simulink model "dc_dc_converter"  (Simulink 7.5)
settings: Solver=ode45  StartTime=0.0  StopTime=10.0  RelTol=1e-3
undefined symbols (not defined in the file): powergui
libraries: powerlib x9
settings Model: Creator=mustafasyyd  LastModifiedBy=mustafasyyd

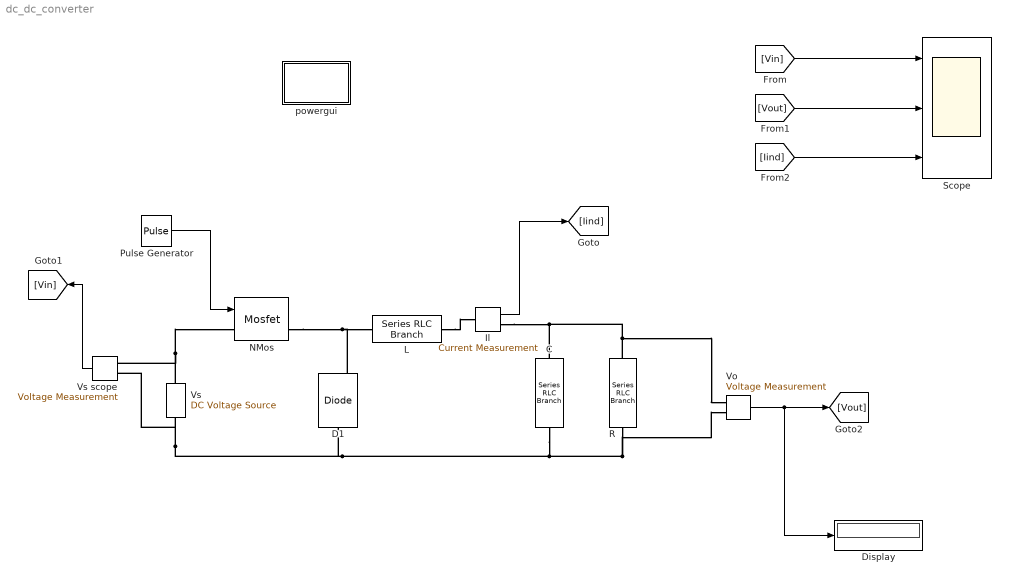
== system dc_dc_converter ==
  C : powerlib/Elements/Series RLC Branch  DialogController=POWERSYS.PowerSysDialog  PhysicalDomain=powersysdomain  SubClassName=unknown  LeftPortType=p1  RightPortType=p1  LConnTagsString=__new0  RConnTagsString=__new0  BranchType=C  Resistance=1  Inductance=1e-3  SetiL0=off  InitialCurrent=0  Capacitance=100e-6  Setx0=off  InitialVoltage=0  Measurements=None
  D1 : powerlib/Power Electronics/Diode  DialogController=POWERSYS.PowerSysDialog  SystemSampleTime=-1  Ron=0.001  Lon=0  Vf=0  IC=0  UseSnubber=off  Rs=500  Cs=250e-9  Measurements=on
  Display : Display
  Il : powerlib/Measurements/Current Measurement  DialogController=POWERSYS.PowerSysDialog  SystemSampleTime=-1  PhasorSimulation=off  OutputType=Complex  PSBequivalent=0
  L : powerlib/Elements/Series RLC Branch  DialogController=POWERSYS.PowerSysDialog  PhysicalDomain=powersysdomain  SubClassName=unknown  LeftPortType=p1  RightPortType=p1  LConnTagsString=__new0  RConnTagsString=__new0  BranchType=L  Resistance=1  Inductance=97.5e-6  SetiL0=off  InitialCurrent=0  Capacitance=1e-6  Setx0=off  InitialVoltage=0  Measurements=None
  NMos : powerlib/Power Electronics/Mosfet  DialogController=POWERSYS.PowerSysDialog  SystemSampleTime=-1  Ron=0.1  Lon=0  Rd=0.01  Vfd=0  IC=0  Rs=1e5  Cs=inf  Measurements=on
  Pulse Generator : DiscretePulseGenerator  PulseType=Time based  Amplitude=1  Period=1/40000  PulseWidth=0.375*100  PhaseDelay=0  SampleTime=1
  R : powerlib/Elements/Series RLC Branch  DialogController=POWERSYS.PowerSysDialog  PhysicalDomain=powersysdomain  SubClassName=unknown  LeftPortType=p1  RightPortType=p1  LConnTagsString=__new0  RConnTagsString=__new0  BranchType=R  Resistance=10  Inductance=0  SetiL0=off  InitialCurrent=0  Capacitance=0  Setx0=off  InitialVoltage=0  Measurements=None
  Scope : Scope  NumInputPorts=3
      settings: TimeRange=10  YMin=48~38.3575~5.55112e-017  YMax=48~38.405~1.3
  Vo : powerlib/Measurements/Voltage Measurement  DialogController=POWERSYS.PowerSysDialog  SystemSampleTime=-1  PhasorSimulation=off  OutputType=Complex  PSBequivalent=0
  Vs : powerlib/Electrical Sources/DC Voltage Source  DialogController=POWERSYS.PowerSysDialog  SystemSampleTime=-1  Amplitude=48  Measurements=None
  Vs scope : powerlib/Measurements/Voltage Measurement  DialogController=POWERSYS.PowerSysDialog  SystemSampleTime=-1  PhasorSimulation=off  OutputType=Complex  PSBequivalent=0
  powergui : Subsystem  Priority=1  AncestorBlock=powerlib/powergui  InitFcn=powergui( 'InitFcn_Callback' , gcb , 0 , [ ] );  StopFcn=powergui( 'StopFcn_Callback' , gcb , 0 , [ ] );  mask(PSB option menu block){SimulationMode=Continuous, SampleTime=50e-6, frequency=60, SPID=off, DisableSnubberDevices=off, DisableRonSwitches=off, DisableVfSwitches=off, SwTol=0, Interpol=off, frequencyindice=0, echomessages=off, HookPort=off, DisplayEquations=off, FunctionMessages=off, EnableUseOfTLC=off, x0status=blocks, RestoreLinks=warning, ResistiveCurrentMeasurement=off, Frange=, Ylog=off, Xlog=on, ShowGrid=off, save=off, variable=ZData, structure=, ZoomFFT=off, StartTime=0.0, cycles=1, DisplayStyle=1, fundamental=, FreqAxis=off, MaxFrequency=1000, frequencyindicesteady=1, RmsSteady=, display=off, Ts=, methode=off}
      mask prompts: SimulationMode "Simulation type:"; SampleTime "Sample time (s):"; frequency "Phasor frequency (Hz):"; SPID "Enable use of ideal switching devices"; DisableSnubberDevices "Disable snubbers in switching devices"; DisableRonSwitches "Disable On resistance in switching devices (Ron=0)"; DisableVfSwitches "Disable Forward voltage in switching devices (Vf=0)"; SwTol "Switch tolerance"; Interpol "Interpolate"; frequencyindice "Load flow frequency (Hz):"; echomessages "Display SimPowerSystems warnings and messages"; HookPort "Add a hook port to the powergui block"; DisplayEquations "Display circuit differential equations"; FunctionMessages "Display internal function messages (debug mode feature)"; EnableUseOfTLC "Use TLC file when in Accelerator Simulation Mode and for RTW applications"; x0status "Start simulation with initial electrical states from:"; RestoreLinks "Restore disabled links of SimPowerSystems blocks:"; ResistiveCurrentMeasurement "Use non ideal current measurement blocks (1e-4Ohm internal resistance)"; Frange "Frequency Range"; Ylog "Log impedance"; Xlog "log Frequency"; ShowGrid "grid"; save "Save Data To Workspace"; variable "Variable Name"; structure "Structure Name (PSBFFTSCOPE)"; ZoomFFT "ZoomFFT (PSBFFTSCOPE)"; StartTime "Start Time (PSBFFTSCOPE)"; cycles "Cycles (PSBFFTSCOPE)"; DisplayStyle "Display style (PSBFFTSCOPE)"; fundamental "Fundamental (PSBFFTSCOPE)"; FreqAxis "Frequency Axis (PSBFFTSCOPE)"; MaxFrequency "Max Frequency (PSBFFTSCOPE)"; frequencyindicesteady "Frequency indice (STEADYSTATE)"; RmsSteady "RMS display (STEADYSTATE)"; display "Display Results"; Ts "Old Ts setting (OBSOLETE)"; methode "Phasor simulation (OBSOLETE)"
      mask help: Set simulation type, simulation parameters, and preferences
      mask init:
      | message = powergui('MaskInitialization',gcb,SimulationMode,SampleTime);
      settings: CopyFcn=powergui( 'Copy_Callback' , gcb , 0 , [ ] );  ModelCloseFcn=powergui( 'CloseButton_Callback' , gcb , [ ] , [ ] );  NameChangeFcn=powergui( 'NameChangeFcn_Callback' , gcb , 0 , [ ] );  OpenFcn=powergui(gcb,'Open')
      settings: DeleteFcn=|
      | powergui( 'Copy_Callback' , gcb , 1 , [ ] );
      | powergui( 'CloseButton_Callback' , gcb , [ ] , [ ] );
      settings: PreSaveFcn=|
      | powergui( 'PreSaveFcn_Callback' , gcb , [ ] , [ ] );
      | powergui( 'CloseButton_Callback' , gcb , [ ] , [ ] );
      mask Help: web(psbhelp)
      mask StyleString: popup(Continuous|Discrete|Phasor),edit,edit,checkbox,checkbox,checkbox,checkbox,edit,checkbox,edit,checkbox,checkbox,checkbox,checkbox,checkbox,popup(blocks|steady|zero),popup(yes|warning|no),checkbox,edit,checkbox,checkbox,checkbox,checkbox,edit,edit,checkbox,edit,edit,edit,edit,checkbox,edit,edit,edit,checkbox,edit,checkbox
      mask CallbackString: powergui('SimulationType',[],[],gcb);|||powergui('SPID',[],[],gcb);||||||||powergui('HookPort',[],[],gcb);|||||||||||||||||||||||||
      mask TabNameString: Solver,Solver,Solver,Solver,Solver,Solver,Solver,Solver,Solver,Preferences,Preferences,Preferences,Solver,Solver,Preferences,Preferences,Preferences,Preferences,Preferences,Preferences,Preferences,Preferences,Preferences,Preferences,Preferences,Preferences,Preferences,Preferences,Preferences,Preferences,Preferences,Preferences,Preferences,Preferences,Preferences,Solver,Solver
      mask Display: color('blue'),disp(message)
  wires:
  Il/1 -> [Iind]
  Pulse Generator/1 -> NMos/1
  Vo/1 -> Display/1, [Vout]
  Vs scope/1 -> [Vin]
  [Iind] -> Scope/3
  [Vout] -> Scope/2
  [Vin] -> Scope/1
  connections:
  R/LConn1 -- C/LConn1 -- Il/RConn1 -- Vo/LConn1
  NMos/RConn1 -- L/LConn1 -- D1/RConn1
  Vs/RConn1 -- NMos/LConn1 -- Vs scope/LConn1
  L/RConn1 -- Il/LConn1
  C/RConn1 -- R/RConn1 -- Vo/LConn2 -- D1/LConn1 -- Vs/LConn1 -- Vs scope/LConn2

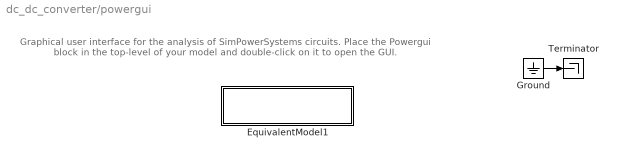
== system dc_dc_converter/powergui ==
  note: Graphical user interface for the analysis of  SimPowerSystems circuits.
      | Place the Powergui block in the top-level of your model and double-click
      | on it to open the GUI.
  EquivalentModel1 : Subsystem
      mask init:
      | S  = GetDataForEquivalentModel('Continuous',gcbh);
      mask Display:
      | color('blue')
      | disp('EQUIVALENT CIRCUIT\nContinuous')
      | disp('')
  Ground : Ground
  Terminator : Terminator
  wires:
  Ground/1 -> Terminator/1

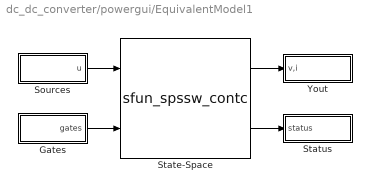
== system dc_dc_converter/powergui/EquivalentModel1 ==
  Gates : Subsystem
  Sources : Subsystem
  State-Space : S-Function  FunctionName=sfun_spssw_contc  Parameters=S.A, S.B, S.C, S.D, S.x0, S.EnableUseOfTLC,S.SwitchResistance ,S.SwitchType, S.SwitchGateInitialValue, S.OutputsToResetToZero  EnableBusSupport=off
  Status : Subsystem
  Yout : Subsystem
  wires:
  Gates/1(gates) -> State-Space/2
  Sources/1(u) -> State-Space/1
  State-Space/2 -> Status/1(status)
  State-Space/1 -> Yout/1(v,i)

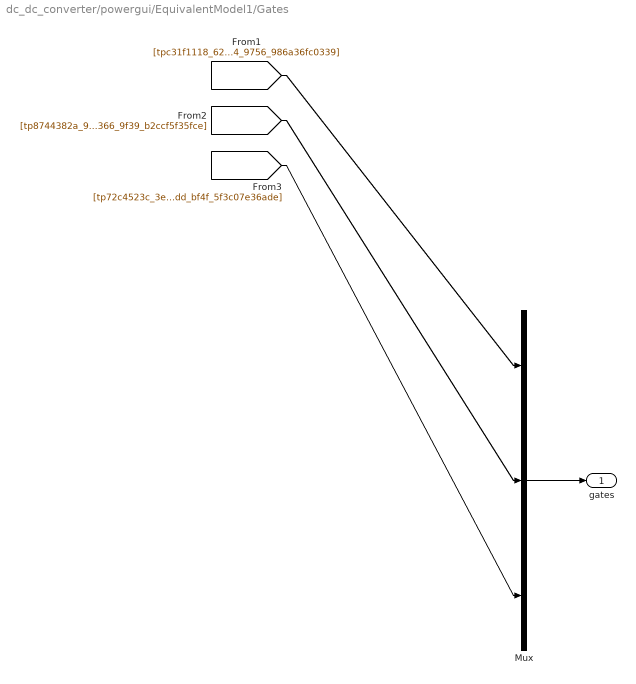
== system dc_dc_converter/powergui/EquivalentModel1/Gates ==
  Mux : Mux  Inputs=[1 1 1]
  gates : Outport  OutDataType=sfix(16)  OutScaling=2^0
  wires:
  Mux/1 -> gates/1
  [tpc31f1118_6209_4864_9756_986a36fc0339] -> Mux/1
  [tp8744382a_9bbe_4366_9f39_b2ccf5f35fce] -> Mux/2
  [tp72c4523c_3edb_46dd_bf4f_5f3c07e36ade] -> Mux/3

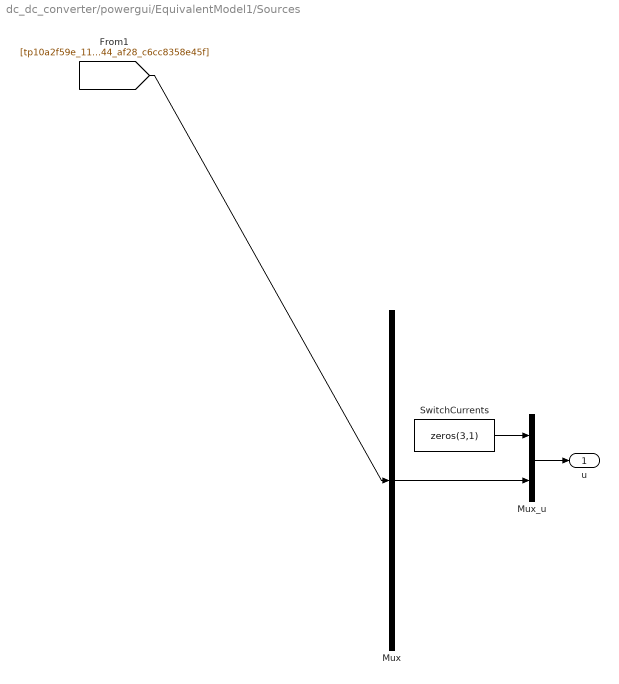
== system dc_dc_converter/powergui/EquivalentModel1/Sources ==
  Mux : Mux  Inputs=1
  Mux_u : Mux  Inputs=[3 1]
  SwitchCurrents : Constant  Value=zeros(3,1)  OutDataType=sfix(16)  OutScaling=2^0
  u : Outport  OutDataType=sfix(16)  OutScaling=2^0
  wires:
  Mux/1 -> Mux_u/2
  SwitchCurrents/1 -> Mux_u/1
  Mux_u/1 -> u/1
  [tp10a2f59e_11f2_4b44_af28_c6cc8358e45f] -> Mux/1

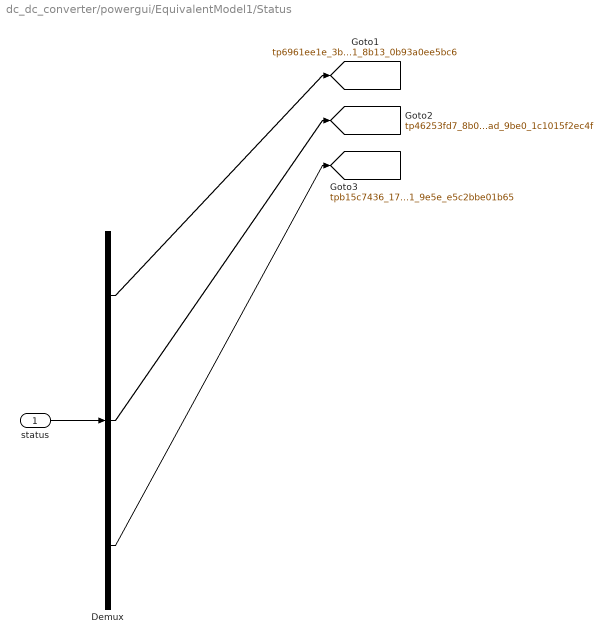
== system dc_dc_converter/powergui/EquivalentModel1/Status ==
  status : Inport  OutDataType=sfix(16)  OutScaling=2^0
  Demux : Demux  Outputs=[1 1 1]
  tag scope: tp46253fd7_8b09_44ad_9be0_1c1015f2ec4f=global, tp6961ee1e_3bec_4761_8b13_0b93a0ee5bc6=global, tpb15c7436_173e_41d1_9e5e_e5c2bbe01b65=global
  wires:
  status/1 -> Demux/1
  Demux/1 -> [tp6961ee1e_3bec_4761_8b13_0b93a0ee5bc6]
  Demux/2 -> [tp46253fd7_8b09_44ad_9be0_1c1015f2ec4f]
  Demux/3 -> [tpb15c7436_173e_41d1_9e5e_e5c2bbe01b65]

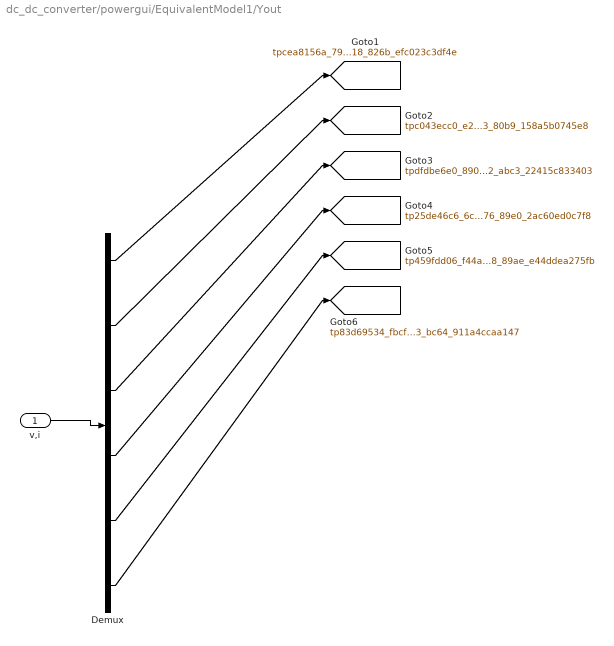
== system dc_dc_converter/powergui/EquivalentModel1/Yout ==
  v,i : Inport  OutDataType=sfix(16)  OutScaling=2^0
  Demux : Demux  Outputs=[1 1 1 1 1 1]
  tag scope: tp25de46c6_6c82_4376_89e0_2ac60ed0c7f8=global, tp459fdd06_f44a_4f98_89ae_e44ddea275fb=global, tp83d69534_fbcf_4753_bc64_911a4ccaa147=global, tpc043ecc0_e25d_4a33_80b9_158a5b0745e8=global, tpcea8156a_7973_4118_826b_efc023c3df4e=global, tpdfdbe6e0_890b_4042_abc3_22415c833403=global
  wires:
  v,i/1 -> Demux/1
  Demux/1 -> [tpcea8156a_7973_4118_826b_efc023c3df4e]
  Demux/2 -> [tpc043ecc0_e25d_4a33_80b9_158a5b0745e8]
  Demux/3 -> [tpdfdbe6e0_890b_4042_abc3_22415c833403]
  Demux/4 -> [tp25de46c6_6c82_4376_89e0_2ac60ed0c7f8]
  Demux/5 -> [tp459fdd06_f44a_4f98_89ae_e44ddea275fb]
  Demux/6 -> [tp83d69534_fbcf_4753_bc64_911a4ccaa147]
